simulink model "matla_1"  (R2017b)
settings: Solver=VariableStepAuto  StartTime=0.0  StopTime=10.0  RelTol=1e-3
settings Model: Creator=ABC  LastModifiedBy=ABC

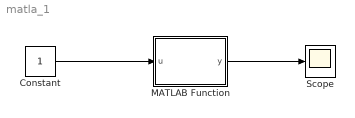
== system matla_1 ==
  Constant : Constant
  MATLAB Function : MATLAB Function  TreatAsAtomicUnit=on
  Scope : Scope
  wires:
  Constant/1 -> MATLAB Function/1(u)
  MATLAB Function/1(y) -> Scope/1

== matlab function matla_1/MATLAB Function ==
  data: u input; y output
function y = fcn(u)

persistent temp 

if isempty(temp), temp = 1; end


if (temp == 0)
    temp = 6;
end

y = temp;
